simulink model "a2_local"  (R2022a)
settings: Solver=FixedStepDiscrete  StartTime=0.0  StopTime=inf  FixedStep=1e-3  RelTol=1e-3  EnableMultiTasking=on
model workspace (MAT data in the model file):
  accel_threhold = 0
undefined symbols (not defined in the file): D0, D1, D10, D11, D12, D13, D2, D3, D4, D5, D6, D7, D8, D9, PTA0, PTA1, PTA2, PTB23, PTB9, PTC16, PTC17, PTC2, PTC3, PTC4, PTD0, PTD1, PTD2, PTD3
libraries: frdmk64flib x17
settings Model: SimulationMode=external  NumberOfSteps=2  ExtModeTrigDuration=5  Creator=Xu Yue  LastModifiedBy=Xu Yue
settings SolverCC: AutoInsertRateTranBlk=on
settings OptimizationCC: EnhancedBackFolding=on  PassReuseOutputArgsAs=Individual arguments  StateBitsets=on  DataBitsets=on  ZeroExternalMemoryAtStartup=off  ZeroInternalMemoryAtStartup=off  NoFixptDivByZeroProtection=on  MaxStackSize=64  OptimizeBlockOrder=speed  DifferentSizesBufferReuse=on  EfficientTunableParamExpr=on
settings DebuggingCC: ParameterTunabilityLossMsg=error
settings HardwareCC: ProdBitPerPointer=32  ProdBitPerSizeT=32  ProdBitPerPtrDiffT=32  ProdLargestAtomicInteger=Long  ProdLargestAtomicFloat=Double  ProdWordSize=32  ProdHWDeviceType=ARM Compatible->ARM Cortex
settings SFSimCC: MATLABDynamicMemAlloc=off
settings RTWCC: SystemTargetFile=ert.tlc  HardwareBoard=NXP FRDM-K64F  TLCOptions="-p0 -aInlineSetEventsForThisBaseRateFcn=TLC_FALSE -aSuppressMultiTaskScheduler=TLC_FALSE  -aRateBasedStepFcn=0"  TemplateMakefile=ert_default_tmf  Toolchain=GNU Tools for ARM Embedded Processors
settings CodeAppCC: ForceParamTrailComments=on  IgnoreCustomStorageClasses=off  OperatorAnnotations=on  SimulinkDataObjDesc=on  SFDataObjDesc=on  InsertBlockDesc=on
settings ERTTargetCC: ExtModeTransport=4  ExtModeMexFile=sendToCommService

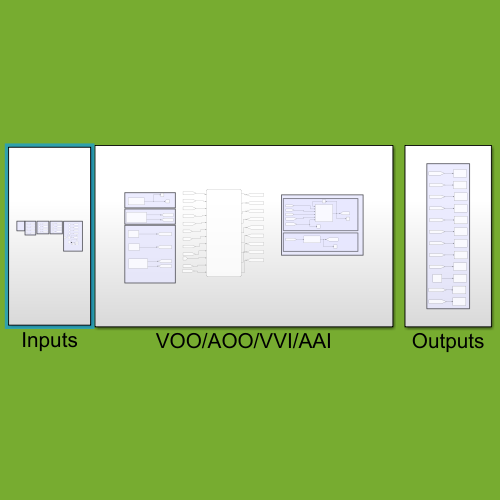
[thumbnail: Simulink's stored preview of the top-level diagram]
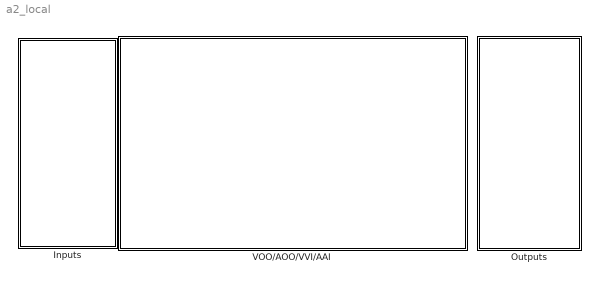
== system a2_local ==
  Inputs : Subsystem
  Outputs : Subsystem
  VOO/AOO/VVI/AAI : Subsystem

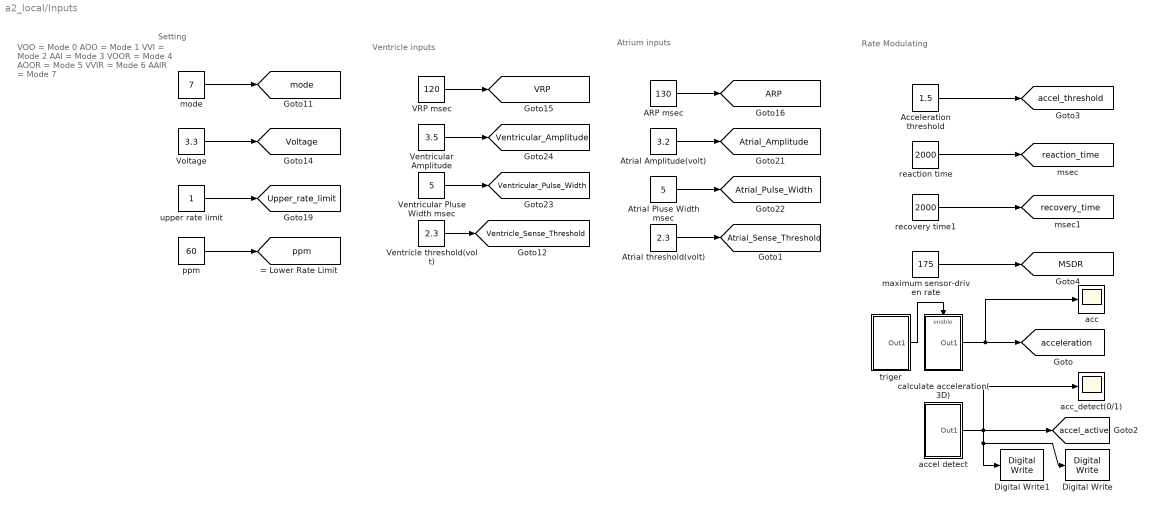
== system a2_local/Inputs ==
  note: Rate Modulating
  note: VOO = Mode 0
      | AOO = Mode 1
      | VVI = Mode 2
      | AAI = Mode 3
      | VOOR = Mode 4
      | AOOR = Mode 5
      | VVIR = Mode 6
      | AAIR = Mode 7
  note: Atrium inputs
  note: Setting
  note: Ventricle inputs
  ARP msec : Constant  Value=130
  Acceleration threshold : Constant  Value=1.5
  Atrial Amplitude(volt) : Constant  Value=3.2
  Atrial Pluse Width msec : Constant  Value=5
  Atrial threshold(volt) : Constant  Value=2.3
  Digital Write : frdmk64flib/Digital Write  Whichpin=GREEN_LED
  Digital Write1 : frdmk64flib/Digital Write  Whichpin=BLUE_LED
  VRP msec : Constant  Value=120
  Ventricle threshold(volt) : Constant  Value=2.3
  Ventricular Amplitude : Constant  Value=3.5
  Ventricular Pluse Width msec : Constant  Value=5
  Voltage : Constant  Value=3.3
  acc : Scope
  acc_detect(0/1) : Scope
  accel detect : Subsystem
  calculate acceleration(3D) : Subsystem
  maximum sensor-driven rate : Constant  Value=175
  mode : Constant  Value=7
  ppm : Constant  Value=60
  reaction time : Constant  Value=2000
  recovery time1 : Constant  Value=2000
  triger : Subsystem
  upper rate limit : Constant
  tag scope: ARP=global, Atrial_Amplitude=global, Atrial_Pulse_Width=global, Atrial_Sense_Threshold=global, MSDR=global, Upper_rate_limit=global, VRP=global, Ventricle_Sense_Threshold=global, Ventricular_Amplitude=global, Ventricular_Pulse_Width=global, Voltage=global, accel_active=global, accel_threshold=global, acceleration=global, mode=global, ppm=global, reaction_time=global, recovery_time=global
  wires:
  Ventricular Pluse Width msec/1 -> [Ventricular_Pulse_Width]
  Voltage/1 -> [Voltage]
  ppm/1 -> [ppm]
  mode/1 -> [mode]
  Ventricular Amplitude/1 -> [Ventricular_Amplitude]
  VRP msec/1 -> [VRP]
  upper rate limit/1 -> [Upper_rate_limit]
  Atrial Pluse Width msec/1 -> [Atrial_Pulse_Width]
  ARP msec/1 -> [ARP]
  Atrial Amplitude(volt)/1 -> [Atrial_Amplitude]
  Atrial threshold(volt)/1 -> [Atrial_Sense_Threshold]
  Ventricle threshold(volt)/1 -> [Ventricle_Sense_Threshold]
  Acceleration threshold/1 -> [accel_threshold]
  calculate acceleration(3D)/1(Out1) -> acc/1, [acceleration]
  accel detect/1(Out1) -> acc_detect(0/1)/1, [accel_active], Digital Write1/1, Digital Write/1
  maximum sensor-driven rate/1 -> [MSDR]
  reaction time/1 -> [reaction_time]
  recovery time1/1 -> [recovery_time]
  triger/1(Out1) -> calculate acceleration(3D)/Enable

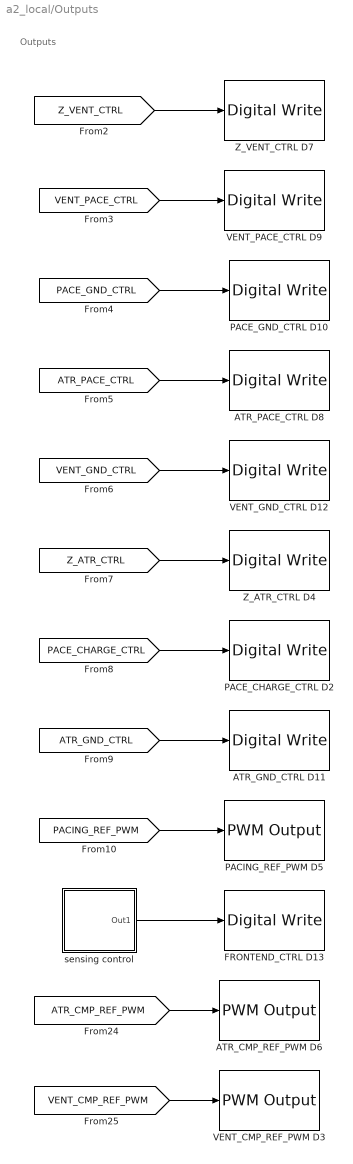
== system a2_local/Outputs ==
  note: Outputs
  ATR_CMP_REF_PWM D6 : frdmk64flib/PWM Output  Whichpin=PTC2 (D6)  InitialFrequency=2000  InitialDutyCycle=0
  ATR_GND_CTRL D11 : frdmk64flib/Digital Write  Whichpin=PTD2 (D11)
  ATR_PACE_CTRL D8 : frdmk64flib/Digital Write  Whichpin=PTA0 (D8)
  FRONTEND_CTRL D13 : frdmk64flib/Digital Write  Whichpin=PTD1 (D13)
  PACE_CHARGE_CTRL D2 : frdmk64flib/Digital Write  Whichpin=PTB9 (D2)
  PACE_GND_CTRL D10 : frdmk64flib/Digital Write  Whichpin=PTD0 (D10)
  PACING_REF_PWM D5 : frdmk64flib/PWM Output  Whichpin=PTA2 (D5)  InitialFrequency=2000  InitialDutyCycle=0
  VENT_CMP_REF_PWM D3 : frdmk64flib/PWM Output  Whichpin=PTA1 (D3)  InitialFrequency=2000  InitialDutyCycle=0
  VENT_GND_CTRL D12 : frdmk64flib/Digital Write  Whichpin=PTD3 (D12)
  "VENT_PACE_CTRL D9  " : frdmk64flib/Digital Write  Whichpin=PTC4 (D9)
  Z_ATR_CTRL D4 : frdmk64flib/Digital Write  Whichpin=PTB23 (D4)
  Z_VENT_CTRL D7 : frdmk64flib/Digital Write  Whichpin=PTC3 (D7)
  sensing control : Subsystem
  wires:
  [VENT_GND_CTRL] -> VENT_GND_CTRL D12/1
  [ATR_PACE_CTRL] -> ATR_PACE_CTRL D8/1
  [PACE_CHARGE_CTRL] -> PACE_CHARGE_CTRL D2/1
  [VENT_PACE_CTRL] -> "VENT_PACE_CTRL D9  "/1
  [Z_VENT_CTRL] -> Z_VENT_CTRL D7/1
  [PACE_GND_CTRL] -> PACE_GND_CTRL D10/1
  [Z_ATR_CTRL] -> Z_ATR_CTRL D4/1
  [PACING_REF_PWM] -> PACING_REF_PWM D5/1
  [ATR_CMP_REF_PWM] -> ATR_CMP_REF_PWM D6/1
  [VENT_CMP_REF_PWM] -> VENT_CMP_REF_PWM D3/1
  [ATR_GND_CTRL] -> ATR_GND_CTRL D11/1
  sensing control/1(Out1) -> FRONTEND_CTRL D13/1

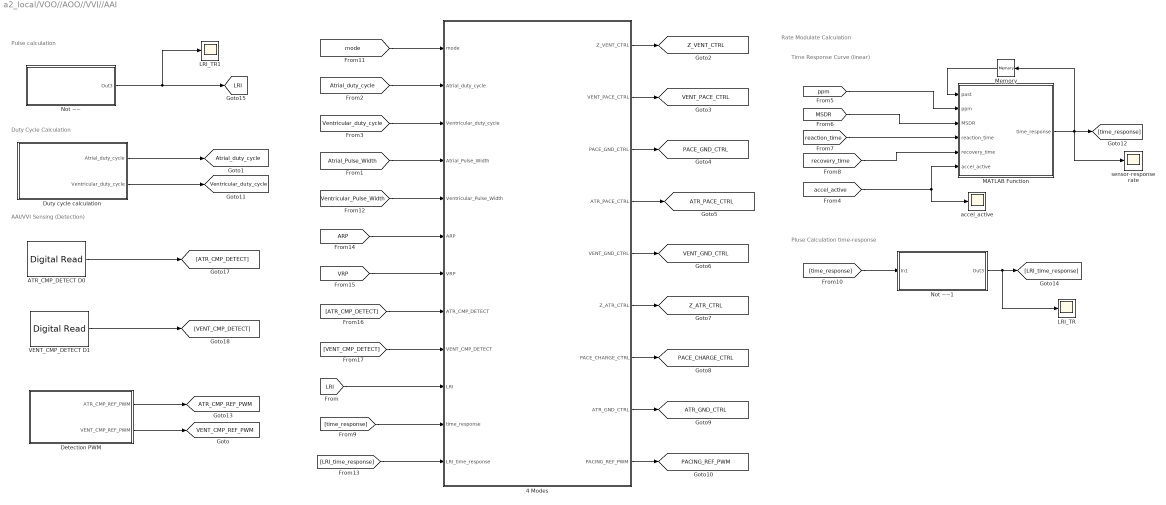
== system a2_local/VOO//AOO//VVI//AAI ==
  note: Pluse Calculation time-response
  note: Time Response Curve (linear)
  note: Rate Modulate Calculation
  note: Duty Cycle Calculation
  note: Pulse calculation
  note: AAI/VVI Sensing (Detection)
  4 Modes : Stateflow chart  TreatAsAtomicUnit=on
      settings: PortSchema="{\"entries\":[{\"content\":{\"sides\":[{\"content\":{\"connectorIds\":[\"In1\",\"In2\",\"In3\",\"In4\",\"In5\",\"In6\",\"In7\",\"In8\",\"In10\",\"In9\",\"In11\",\"In12\"]},\"type\":\"ConnectorPlacement.EquallySpacedRectSide\",\"uuid\":\"cda6f2b2-e06a-45ee-a605-83fcbb92a490\"},{\"content\":{\"connectorIds\":[\"Out1\",\"Out2\",\"Out3\",\"Out4\",\"Out5\",\"Out6\",\"Out7\",\"Out8\",\"Out9\"],\"side\":\"RIGHT\"},\"type\":\"ConnectorPlacement.EquallySpacedRectSide\",\"uuid\":\"bbaec7b2-cf34-4072-a5a1-e7338d619e1a\"},{\"content\":{\"connectorIds\":[],\"side\":\"TOP\"},\"type\":\"ConnectorPlacement.EquallySpacedRectSide\",\"uuid\":\"0d445168-f6f3-41dc-a420-b501484e0774\"},{\"content\":{\"connectorIds\":[],\"side\":\"BOTTOM\"},\"type\":\"ConnectorPlacement.EquallySpacedRectSide\",\"uuid\":\"746170fa-1649-4f06-a75d-d55dc9bad7cc\"}]},\"type\":\"ConnectorPlacement.EquallySpacedConnector\",\"uuid\":\"5da4eaab-cd7d-4de3-80b7-75ac7c893a27\"}],\"packageUris\":[\"http://schema.mathworks.com/mf0/Connector/R2020b\"],\"version\":\"1.0\"}"
  ATR_CMP_DETECT D0 : frdmk64flib/Digital Read  Whichpin=PTC16 (D0)  SampleTime=-1
  Detection PWM : Subsystem
  Duty cycle calculation : Subsystem
  LRI_TR : Scope
  LRI_TR1 : Scope
  MATLAB Function : MATLAB Function  TreatAsAtomicUnit=on
  Memory : Memory
  Not ~~ : Subsystem
  Not ~~1 : Subsystem
  VENT_CMP_DETECT D1 : frdmk64flib/Digital Read  Whichpin=PTC17 (D1)  SampleTime=-1
  accel_active : Scope
  sensor-response rate : Scope
  tag scope: ATR_CMP_REF_PWM=global, ATR_GND_CTRL=global, ATR_PACE_CTRL=global, Atrial_duty_cycle=global, LRI=global, PACE_CHARGE_CTRL=global, PACE_GND_CTRL=global, PACING_REF_PWM=global, VENT_CMP_REF_PWM=global, VENT_GND_CTRL=global, VENT_PACE_CTRL=global, Ventricular_duty_cycle=global, Z_ATR_CTRL=global, Z_VENT_CTRL=global
  wires:
  4 Modes/5(VENT_GND_CTRL) -> [VENT_GND_CTRL]
  4 Modes/1(Z_VENT_CTRL) -> [Z_VENT_CTRL]
  4 Modes/8(ATR_GND_CTRL) -> [ATR_GND_CTRL]
  Detection PWM/1(ATR_CMP_REF_PWM) -> [ATR_CMP_REF_PWM]
  [mode] -> 4 Modes/1(mode)
  4 Modes/6(Z_ATR_CTRL) -> [Z_ATR_CTRL]
  4 Modes/3(PACE_GND_CTRL) -> [PACE_GND_CTRL]
  4 Modes/9(PACING_REF_PWM) -> [PACING_REF_PWM]
  [ATR_CMP_DETECT] -> 4 Modes/8(ATR_CMP_DETECT)
  4 Modes/2(VENT_PACE_CTRL) -> [VENT_PACE_CTRL]
  ATR_CMP_DETECT D0/1 -> [ATR_CMP_DETECT]
  [VENT_CMP_DETECT] -> 4 Modes/10(VENT_CMP_DETECT)
  [Atrial_Pulse_Width] -> 4 Modes/4(Atrial_Pulse_Width)
  [ARP] -> 4 Modes/6(ARP)
  [Ventricular_Pulse_Width] -> 4 Modes/5(Ventricular_Pulse_Width)
  4 Modes/4(ATR_PACE_CTRL) -> [ATR_PACE_CTRL]
  [VRP] -> 4 Modes/7(VRP)
  4 Modes/7(PACE_CHARGE_CTRL) -> [PACE_CHARGE_CTRL]
  Detection PWM/2(VENT_CMP_REF_PWM) -> [VENT_CMP_REF_PWM]
  Duty cycle calculation/1(Atrial_duty_cycle) -> [Atrial_duty_cycle]
  Duty cycle calculation/2(Ventricular_duty_cycle) -> [Ventricular_duty_cycle]
  [Atrial_duty_cycle] -> 4 Modes/2(Atrial_duty_cycle)
  [Ventricular_duty_cycle] -> 4 Modes/3(Ventricular_duty_cycle)
  VENT_CMP_DETECT D1/1 -> [VENT_CMP_DETECT]
  Not ~~/1(Out3) -> LRI_TR1/1, [LRI]
  [LRI] -> 4 Modes/9(LRI)
  [MSDR] -> MATLAB Function/3(MSDR)
  [accel_active] -> accel_active/1, MATLAB Function/6(accel_active)
  [recovery_time] -> MATLAB Function/5(recovery_time)
  [ppm] -> MATLAB Function/2(ppm)
  [reaction_time] -> MATLAB Function/4(reaction_time)
  MATLAB Function/1(time_response) -> [time_response], Memory/1, sensor-response rate/1
  Memory/1 -> MATLAB Function/1(past)
  [time_response] -> 4 Modes/11(time_response)
  [time_response] -> Not ~~1/1(In1)
  Not ~~1/1(Out3) -> LRI_TR/1, [LRI_time_response]
  [LRI_time_response] -> 4 Modes/12(LRI_time_response)

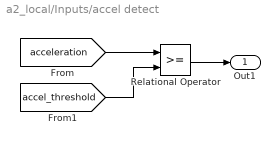
== system a2_local/Inputs/accel detect ==
  Relational Operator : RelationalOperator  OutDataTypeStr=boolean  RndMeth=Simplest  InputSameDT=off
  Out1 : Outport
  wires:
  [accel_threshold] -> Relational Operator/2
  [acceleration] -> Relational Operator/1
  Relational Operator/1 -> Out1/1

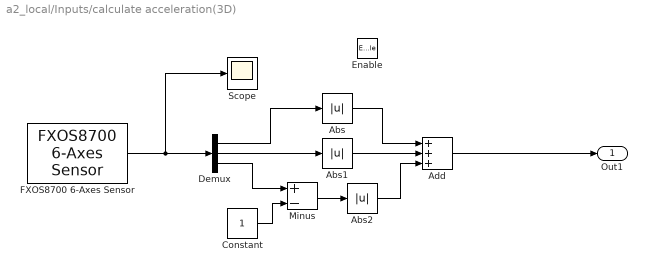
== system a2_local/Inputs/calculate acceleration(3D) ==
  Enable : EnablePort
  Abs : Abs  SaturateOnIntegerOverflow=off
  Abs1 : Abs  SaturateOnIntegerOverflow=off
  Abs2 : Abs  SaturateOnIntegerOverflow=off
  Add : Sum  Inputs=+++
  Constant : Constant
  Demux : Demux  Outputs=3
  FXOS8700 6-Axes Sensor : frdmk64flib/FXOS8700 6-Axes Sensor  Activesensor=Accelerometer only  ODR=100Hz  HybridODR=400Hz  Accelfullrange=-4g to +4g  SampleTime=-1
  Minus : Sum  Inputs=+-
  Scope : Scope
  Out1 : Outport
  wires:
  Abs1/1 -> Add/2
  Abs2/1 -> Add/3
  Demux/1 -> Abs/1
  FXOS8700 6-Axes Sensor/1 -> Scope/1, Demux/1
  Abs/1 -> Add/1
  Minus/1 -> Abs2/1
  Demux/2 -> Abs1/1
  Demux/3 -> Minus/1
  Constant/1 -> Minus/2
  Add/1 -> Out1/1

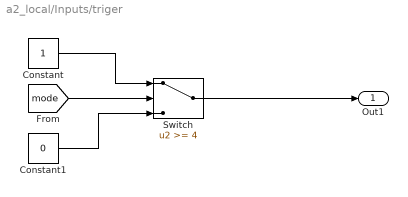
== system a2_local/Inputs/triger ==
  Constant : Constant
  Constant1 : Constant  Value=0
  Switch : Switch  Threshold=4  SaturateOnIntegerOverflow=off  InputSameDT=off
  Out1 : Outport
  wires:
  Constant/1 -> Switch/1
  [mode] -> Switch/2
  Constant1/1 -> Switch/3
  Switch/1 -> Out1/1

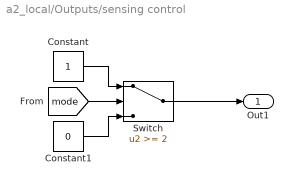
== system a2_local/Outputs/sensing control ==
  Constant : Constant
  Constant1 : Constant  Value=0
  Switch : Switch  Threshold=2  SaturateOnIntegerOverflow=off  InputSameDT=off
  Out1 : Outport
  wires:
  Constant/1 -> Switch/1
  Constant1/1 -> Switch/3
  [mode] -> Switch/2
  Switch/1 -> Out1/1

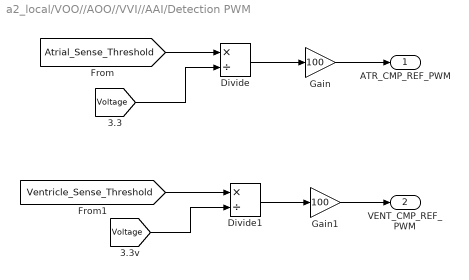
== system a2_local/VOO//AOO//VVI//AAI/Detection PWM ==
  Divide : Product  Inputs=*/  RndMeth=Zero  SaturateOnIntegerOverflow=on
  Divide1 : Product  Inputs=*/  RndMeth=Zero  SaturateOnIntegerOverflow=on
  Gain : Gain  Gain=100
  Gain1 : Gain  Gain=100
  ATR_CMP_REF_PWM : Outport
  VENT_CMP_REF_PWM : Outport  Port=2
  wires:
  Divide/1 -> Gain/1
  Gain/1 -> ATR_CMP_REF_PWM/1
  [Voltage] -> Divide1/2
  Divide1/1 -> Gain1/1
  Gain1/1 -> VENT_CMP_REF_PWM/1
  [Voltage] -> Divide/2
  [Atrial_Sense_Threshold] -> Divide/1
  [Ventricle_Sense_Threshold] -> Divide1/1

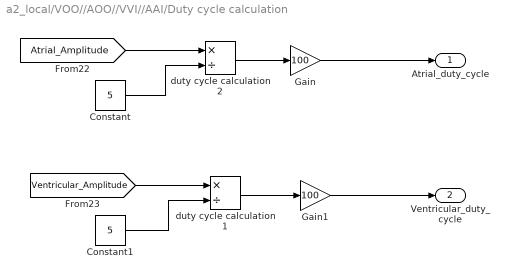
== system a2_local/VOO//AOO//VVI//AAI/Duty cycle calculation ==
  Constant : Constant  Value=5
  Constant1 : Constant  Value=5
  Gain : Gain  Gain=100
  Gain1 : Gain  Gain=100
  duty cycle calculation1 : Product  Inputs=*/  RndMeth=Zero  SaturateOnIntegerOverflow=on
  duty cycle calculation2 : Product  Inputs=*/  RndMeth=Zero  SaturateOnIntegerOverflow=on
  Atrial_duty_cycle : Outport
  Ventricular_duty_cycle : Outport  Port=2
  wires:
  Gain/1 -> Atrial_duty_cycle/1
  Gain1/1 -> Ventricular_duty_cycle/1
  duty cycle calculation1/1 -> Gain1/1
  duty cycle calculation2/1 -> Gain/1
  Constant1/1 -> duty cycle calculation1/2
  Constant/1 -> duty cycle calculation2/2
  [Ventricular_Amplitude] -> duty cycle calculation1/1
  [Atrial_Amplitude] -> duty cycle calculation2/1

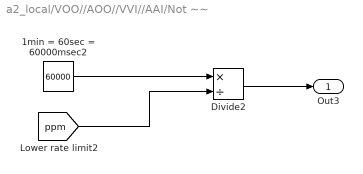
== system a2_local/VOO//AOO//VVI//AAI/Not ~~ ==
  1min = 60sec = 60000msec2 : Constant  Value=60000
  Divide2 : Product  Inputs=*/
  Out3 : Outport
  wires:
  [ppm] -> Divide2/2
  1min = 60sec = 60000msec2/1 -> Divide2/1
  Divide2/1 -> Out3/1

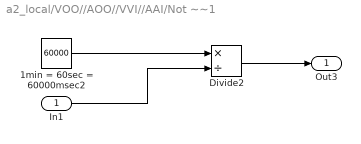
== system a2_local/VOO//AOO//VVI//AAI/Not ~~1 ==
  In1 : Inport
  1min = 60sec = 60000msec2 : Constant  Value=60000
  Divide2 : Product  Inputs=*/
  Out3 : Outport
  wires:
  Divide2/1 -> Out3/1
  1min = 60sec = 60000msec2/1 -> Divide2/1
  In1/1 -> Divide2/2

== matlab function a2_local/VOO//AOO//VVI//AAI/MATLAB Function ==
  data: past input; ppm input; time_response output; MSDR input; reaction_time input; recovery_time input; accel_active input
function time_response = fcn(past, ppm, MSDR, reaction_time, recovery_time, accel_active)

%assuming all linear increase & decrease
pos_slope = (MSDR - ppm) / reaction_time;
neg_slope = -(MSDR - ppm) / recovery_time;

t_step = 1; %msec
if past == 0
    current = ppm;
else
    current = past;
end

%active
if accel_active == 1
    current = current + pos_slope*t_step;
    if current > MSDR
        current = MSDR;
    end

%disactive
else
    current = current + neg_slope*t_step;
    if current < ppm
        current = ppm;
    end
end

time_response=current;

== stateflow chart a2_local/VOO//AOO//VVI//AAI/4 Modes ==
  state VOOR
    state VOOR [group]
      state Charging
        entry:
        %Charging C22
        ATR_PACE_CTRL = LOW
        VENT_PACE_CTRL = LOW
        PACING_REF_PWM = Ventricular_duty_cycle
        PACE_CHARGE_CTRL = HIGH
        %Discharging Blocking Cap C21
        PACE_GND_CTRL = HIGH
        VENT_PACE_CTRL = LOW
        Z_ATR_CTRL = LOW
        Z_VENT_CTRL = LOW
        ATR_PACE_CTRL = LOW
        ATR_GND_CTRL = LOW
        VENT_GND_CTRL = HIGH
      state Pacing
        entry:
        %Discharge C22 (Charge C21)
        PACE_CHARGE_CTRL = LOW
        PACE_GND_CTRL = HIGH
        ATR_PACE_CTRL = LOW
        ATR_GND_CTRL = LOW
        Z_ATR_CTRL = LOW
        Z_VENT_CTRL = LOW
        VENT_GND_CTRL = LOW
        VENT_PACE_CTRL = HIGH
      VOOR.VOOR.Charging -> VOOR.VOOR.Pacing [order 2] : [after(0.5*LRI_time_response-Ventricular_Pulse_Width,msec)]
      VOOR.VOOR.Pacing -> VOOR.VOOR.Charging : [after(Ventricular_Pulse_Width,msec)]
  state AOOR
    state AOOR [group]
      state Charging
        entry:
        %Charging C22
        ATR_PACE_CTRL = LOW
        VENT_PACE_CTRL = LOW
        PACING_REF_PWM = Atrial_duty_cycle
        PACE_CHARGE_CTRL = HIGH
        %Discharging Blocking Cap C21
        PACE_GND_CTRL = HIGH
        VENT_PACE_CTRL = LOW
        Z_ATR_CTRL = LOW
        Z_VENT_CTRL = LOW
        ATR_PACE_CTRL = LOW
        ATR_GND_CTRL = HIGH
        VENT_GND_CTRL = LOW
      state Pacing
        entry:
        %Discharge C22 (Charge C21)
        PACE_CHARGE_CTRL = LOW
        PACE_GND_CTRL = HIGH
        ATR_PACE_CTRL = HIGH
        ATR_GND_CTRL = LOW
        Z_ATR_CTRL = LOW
        Z_VENT_CTRL = LOW
        VENT_GND_CTRL = LOW
        VENT_PACE_CTRL = LOW
      AOOR.AOOR.Charging -> AOOR.AOOR.Pacing [order 1] : after(0.5*LRI_time_response-Atrial_Pulse_Width,msec)
      AOOR.AOOR.Pacing -> AOOR.AOOR.Charging : after(Atrial_Pulse_Width,msec)
  state VVIR
    state VVIR [group]
      state Pacing
        entry:
        %Discharge C22 (Charge C21)
        PACE_CHARGE_CTRL = LOW
        PACE_GND_CTRL = HIGH
        ATR_PACE_CTRL = LOW
        ATR_GND_CTRL = LOW
        Z_ATR_CTRL = LOW
        Z_VENT_CTRL = LOW
        VENT_GND_CTRL = LOW
        VENT_PACE_CTRL = HIGH
      state Charging
        entry:
        %Charging C22
        ATR_PACE_CTRL = LOW
        VENT_PACE_CTRL = LOW
        PACING_REF_PWM = Ventricular_duty_cycle
        PACE_CHARGE_CTRL = HIGH
        %Discharging Blocking Cap C21
        PACE_GND_CTRL = HIGH
        VENT_PACE_CTRL = LOW
        Z_ATR_CTRL = LOW
        Z_VENT_CTRL = LOW
        ATR_PACE_CTRL = LOW
        ATR_GND_CTRL = LOW
        VENT_GND_CTRL = HIGH
      state VRP_Period
        %refactory period
      state Alert_Period
        %If nature pace occur
        %go back to VRP_Period
      VVIR.VVIR.Alert_Period -> VVIR.VVIR.VRP_Period [order 1] : [VENT_CMP_DETECT ==  true]
      VVIR.VVIR.VRP_Period -> VVIR.VVIR.Alert_Period : after(VRP, msec)
      VVIR.VVIR.Alert_Period -> VVIR.VVIR.Pacing [order 2] : after(0.5*LRI_time_response-Ventricular_Pulse_Width-VRP,msec)
      VVIR.VVIR.Charging -> VVIR.VVIR.Alert_Period [order 1] : after(VRP, msec)
      VVIR.VVIR.Pacing -> VVIR.VVIR.Charging : after(Ventricular_Pulse_Width,msec)
  state AAIR
    state AAIR [group]
      state Alert_Period
        %If nature pace occur
        %reset ARP_Period
      state ARP_Period
        %refractory period
      state Charging
        entry:
        %Charging C22
        ATR_PACE_CTRL = LOW
        VENT_PACE_CTRL = LOW
        PACING_REF_PWM = Atrial_duty_cycle
        PACE_CHARGE_CTRL = HIGH
        %Discharging Blocking Cap C21
        PACE_GND_CTRL = HIGH
        VENT_PACE_CTRL = LOW
        Z_ATR_CTRL = LOW
        Z_VENT_CTRL = LOW
        ATR_PACE_CTRL = LOW
        ATR_GND_CTRL = HIGH
        VENT_GND_CTRL = LOW
      state Pacing
        entry:
        %Discharge C22 (Charge C21)
        PACE_CHARGE_CTRL = LOW
        PACE_GND_CTRL = HIGH
        ATR_PACE_CTRL = HIGH
        ATR_GND_CTRL = LOW
        Z_ATR_CTRL = LOW
        Z_VENT_CTRL = LOW
        VENT_GND_CTRL = LOW
        VENT_PACE_CTRL = LOW
      AAIR.AAIR.Alert_Period -> AAIR.AAIR.ARP_Period [order 1] : [ATR_CMP_DETECT == true]
      AAIR.AAIR.Alert_Period -> AAIR.AAIR.Pacing [order 2] : after(0.5*LRI_time_response-Atrial_Pulse_Width-ARP, msec)
      AAIR.AAIR.ARP_Period -> AAIR.AAIR.Alert_Period : after(ARP, msec)
      AAIR.AAIR.Charging -> AAIR.AAIR.Alert_Period [order 1] : after(ARP, msec)
      AAIR.AAIR.Pacing -> AAIR.AAIR.Charging : after(Atrial_Pulse_Width, msec)
  state VOO
    state VOO [group]
      state Charging
        entry:
        %Charging C22
        ATR_PACE_CTRL = LOW
        VENT_PACE_CTRL = LOW
        PACING_REF_PWM = Ventricular_duty_cycle
        PACE_CHARGE_CTRL = HIGH
        %Discharging Blocking Cap C21
        PACE_GND_CTRL = HIGH
        VENT_PACE_CTRL = LOW
        Z_ATR_CTRL = LOW
        Z_VENT_CTRL = LOW
        ATR_PACE_CTRL = LOW
        ATR_GND_CTRL = LOW
        VENT_GND_CTRL = HIGH
      state Pacing
        entry:
        %Discharge C22 (Charge C21)
        PACE_CHARGE_CTRL = LOW
        PACE_GND_CTRL = HIGH
        ATR_PACE_CTRL = LOW
        ATR_GND_CTRL = LOW
        Z_ATR_CTRL = LOW
        Z_VENT_CTRL = LOW
        VENT_GND_CTRL = LOW
        VENT_PACE_CTRL = HIGH
      VOO.VOO.Charging -> VOO.VOO.Pacing [order 2] : [after(LRI-Ventricular_Pulse_Width,msec)]
      VOO.VOO.Pacing -> VOO.VOO.Charging : [after(Ventricular_Pulse_Width,msec)]
  state Start
    % mode 0 = VOO
    % mode 1 = AOO
    % mode 2 = VVI
    % mode 3 = AAI
  state AOO
    state AOO [group]
      state Charging
        entry:
        %Charging C22
        ATR_PACE_CTRL = LOW
        VENT_PACE_CTRL = LOW
        PACING_REF_PWM = Atrial_duty_cycle
        PACE_CHARGE_CTRL = HIGH
        %Discharging Blocking Cap C21
        PACE_GND_CTRL = HIGH
        VENT_PACE_CTRL = LOW
        Z_ATR_CTRL = LOW
        Z_VENT_CTRL = LOW
        ATR_PACE_CTRL = LOW
        ATR_GND_CTRL = HIGH
        VENT_GND_CTRL = LOW
      state Pacing
        entry:
        %Discharge C22 (Charge C21)
        PACE_CHARGE_CTRL = LOW
        PACE_GND_CTRL = HIGH
        ATR_PACE_CTRL = HIGH
        ATR_GND_CTRL = LOW
        Z_ATR_CTRL = LOW
        Z_VENT_CTRL = LOW
        VENT_GND_CTRL = LOW
        VENT_PACE_CTRL = LOW
      AOO.AOO.Charging -> AOO.AOO.Pacing [order 1] : after(LRI-Atrial_Pulse_Width,msec)
      AOO.AOO.Pacing -> AOO.AOO.Charging : after(Atrial_Pulse_Width,msec)
  state VVI
    state VVI [group]
      state Pacing
        entry:
        %Discharge C22 (Charge C21)
        PACE_CHARGE_CTRL = LOW
        PACE_GND_CTRL = HIGH
        ATR_PACE_CTRL = LOW
        ATR_GND_CTRL = LOW
        Z_ATR_CTRL = LOW
        Z_VENT_CTRL = LOW
        VENT_GND_CTRL = LOW
        VENT_PACE_CTRL = HIGH
      state Charging1
        entry:
        %Charging C22
        ATR_PACE_CTRL = LOW
        VENT_PACE_CTRL = LOW
        PACING_REF_PWM = Ventricular_duty_cycle
        PACE_CHARGE_CTRL = HIGH
        %Discharging Blocking Cap C21
        PACE_GND_CTRL = HIGH
        VENT_PACE_CTRL = LOW
        Z_ATR_CTRL = LOW
        Z_VENT_CTRL = LOW
        ATR_PACE_CTRL = LOW
        ATR_GND_CTRL = LOW
        VENT_GND_CTRL = HIGH
      state VRP_Period
        %refactory period
      state Alert_Period
        %If nature pace occur
        %go back to VRP_Period
      VVI.VVI.Alert_Period -> VVI.VVI.VRP_Period [order 1] : [VENT_CMP_DETECT ==  true]
      VVI.VVI.VRP_Period -> VVI.VVI.Alert_Period : after(VRP, msec)
      VVI.VVI.Alert_Period -> VVI.VVI.Pacing [order 2] : after(LRI-VRP,msec)
      Charging1 -> VVI.VVI.Alert_Period [order 1] : after(VRP, msec)
      VVI.VVI.Pacing -> Charging1 : after(Ventricular_Pulse_Width,msec)
  state AAI
    state AAI [group]
      state Alert_Period
        %If nature pace occur
        %reset ARP_Period
      state ARP_Period
        %refractory period
      state Charging
        entry:
        %Charging C22
        ATR_PACE_CTRL = LOW
        VENT_PACE_CTRL = LOW
        PACING_REF_PWM = Atrial_duty_cycle
        PACE_CHARGE_CTRL = HIGH
        %Discharging Blocking Cap C21
        PACE_GND_CTRL = HIGH
        VENT_PACE_CTRL = LOW
        Z_ATR_CTRL = LOW
        Z_VENT_CTRL = LOW
        ATR_PACE_CTRL = LOW
        ATR_GND_CTRL = HIGH
        VENT_GND_CTRL = LOW
      state Pacing
        entry:
        %Discharge C22 (Charge C21)
        PACE_CHARGE_CTRL = LOW
        PACE_GND_CTRL = HIGH
        ATR_PACE_CTRL = HIGH
        ATR_GND_CTRL = LOW
        Z_ATR_CTRL = LOW
        Z_VENT_CTRL = LOW
        VENT_GND_CTRL = LOW
        VENT_PACE_CTRL = LOW
      AAI.AAI.Alert_Period -> AAI.AAI.ARP_Period [order 1] : [ATR_CMP_DETECT == true]
      AAI.AAI.Alert_Period -> AAI.AAI.Pacing [order 2] : after(LRI - ARP, msec)
      AAI.AAI.ARP_Period -> AAI.AAI.Alert_Period : after(ARP, msec)
      AAI.AAI.Charging -> AAI.AAI.Alert_Period [order 1] : after(ARP, msec)
      AAI.AAI.Pacing -> AAI.AAI.Charging : after(Atrial_Pulse_Width, msec)
  Start -> AAIR.AAIR.Charging [order 8] : [mode == 7]
  Start -> VOOR.VOOR.Charging [order 3] : [mode == 4 ]
  Start -> VVIR.VVIR.Charging [order 7] : [mode == 6]
  Start -> AOOR.AOOR.Charging [order 1] : [mode == 5]
  VOOR.VOOR.Charging -> Start [order 1] : [mode ~= 4]
  AAIR.AAIR.Charging -> Start [order 2] : [mode ~= 7]
  AOOR.AOOR.Charging -> Start [order 2] : [mode ~= 5]
  VVIR.VVIR.Charging -> Start [order 2] : [mode ~= 6]
  (default) -> Start
  AOO.AOO.Charging -> Start [order 2] : [mode ~= 1]
  Charging1 -> Start [order 2] : [mode ~= 2]
  AAI.AAI.Charging -> Start [order 2] : [mode ~= 3]
  VOO.VOO.Charging -> Start [order 1] : [mode ~= 0]
  Start -> VOO.VOO.Charging [order 2] : [mode == 0]
  Start -> AOO.AOO.Charging [order 4] : [mode == 1]
  Start -> AAI.AAI.Charging [order 6] : [mode == 3]
  Start -> Charging1 [order 5] : [mode == 2]
  data: mode input; Z_VENT_CTRL output; VENT_PACE_CTRL output; PACE_GND_CTRL output; ATR_PACE_CTRL output; VENT_GND_CTRL output; Z_ATR_CTRL output; PACE_CHARGE_CTRL output; ATR_GND_CTRL output; PACING_REF_PWM output; LOW constant boolean =0; HIGH constant boolean =1; Atrial_duty_cycle input; Ventricular_duty_cycle input; Atrial_Pulse_Width input; Ventricular_Pulse_Width input; ARP input; VRP input; ATR_CMP_DETECT input; LRI input; VENT_CMP_DETECT input; time_response input; LRI_time_response input
